simulink model "ReformerSpaceTime"  (R2021a)
settings: Solver=ode23tb  StartTime=0.0  StopTime=10000  RelTol=1e-3
values from neighbouring files (symbols this model uses):
  c0 = zeros(Nx,1)    [init_ReformerSpaceTime.m]
  Nx = 25    [init_ReformerSpaceTime.m]
  p = []    [init_ReformerSpaceTime.m]
settings Model: Creator=djoroya  LastModifiedBy=djoroya
settings DebuggingCC: UnconnectedInputMsg=none  UnconnectedOutputMsg=none  UnconnectedLineMsg=none

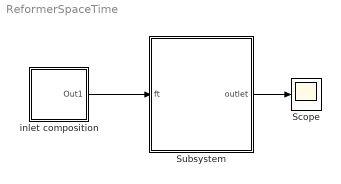
== system ReformerSpaceTime ==
  Scope : Scope
  Subsystem : Subsystem
  inlet composition : Subsystem
  wires:
  inlet composition/1(Out1) -> Subsystem/1(ft)
  Subsystem/1(outlet) -> Scope/1

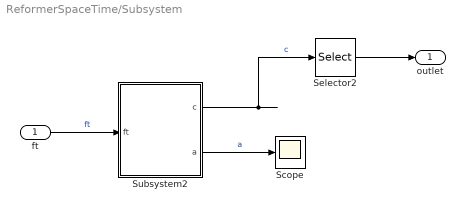
== system ReformerSpaceTime/Subsystem ==
  ft : Inport
  Scope : Scope
  Selector2 : Selector  NumberOfDimensions=2  InputPortWidth=2  IndexOptions=Index vector (dialog),Select all  Indices=Nx,1  OutputSizes=1,1
  Subsystem2 : Subsystem
  outlet : Outport
  wires:
  ft/1 -> Subsystem2/1(ft)  "ft"
  Subsystem2/2(a) -> Scope/1  "a"
  Subsystem2/1(c) -> Selector2/1  "c"
  Selector2/1 -> outlet/1

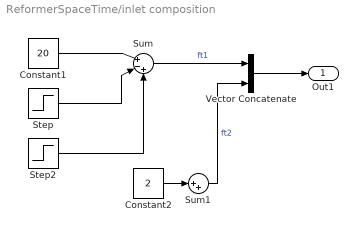
== system ReformerSpaceTime/inlet composition ==
  Constant1 : Constant  Value=20
  Constant2 : Constant  Value=2
  Step : Step  Time=6000  After=20  SampleTime=0
  Step2 : Step  Time=3000  After=10  SampleTime=0
  Sum : Sum  Inputs=|+-+
  Sum1 : Sum  Inputs=|++
  Vector Concatenate : Concatenate  Mode=Multidimensional array  ConcatenateDimension=2
  Out1 : Outport
  wires:
  Constant1/1 -> Sum/1
  Constant2/1 -> Sum1/1
  Sum1/1 -> Vector Concatenate/2  "ft2"
  Sum/1 -> Vector Concatenate/1  "ft1"
  Vector Concatenate/1 -> Out1/1
  Step/1 -> Sum/2
  Step2/1 -> Sum/3

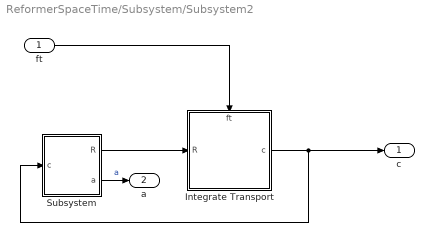
== system ReformerSpaceTime/Subsystem/Subsystem2 ==
  ft : Inport
  Integrate Transport : Subsystem
      settings: PortSchema="{\"entries\":[{\"content\":{\"sides\":[{\"content\":{\"connectorIds\":[\"In1\"]},\"type\":\"ConnectorPlacement.EquallySpacedRectSide\",\"uuid\":\"e3e01424-637b-4a00-a2de-d40794d2ff76\"},{\"content\":{\"connectorIds\":[\"Out1\"],\"side\":\"RIGHT\"},\"type\":\"ConnectorPlacement.EquallySpacedRectSide\",\"uuid\":\"276261e1-850f-4b68-9985-ea5629fd55a5\"},{\"content\":{\"connectorIds\":[\"In2\"],\"side\":\"TOP\"},\"type\":\"ConnectorPlacement.EquallySpacedRectSide\",\"uuid\":\"07b53658-fce3-4297-a7f0-8888709701c4\"}]},\"type\":\"ConnectorPlacement.EquallySpacedConnector\",\"uuid\":\"2f7db6b4-a935-4b8f-9ad3-e9b0cbcdf802\"}],\"packageUris\":[\"http://schema.mathworks.com/mf0/Connector/R2020b\"],\"version\":\"1.0\"}"
  Subsystem : Subsystem
  c : Outport
  a : Outport  Port=2
  wires:
  Subsystem/2(a) -> a/1  "a"
  Subsystem/1(R) -> Integrate Transport/1(R)
  ft/1 -> Integrate Transport/2(ft)
  Integrate Transport/1(c) -> Subsystem/1(c), c/1

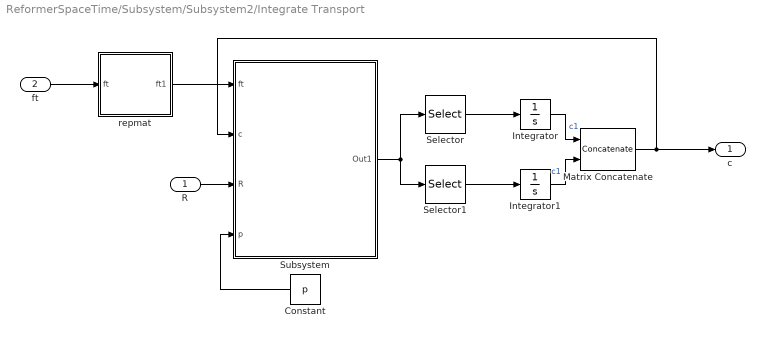
== system ReformerSpaceTime/Subsystem/Subsystem2/Integrate Transport ==
  R : Inport
  ft : Inport  Port=2
  Constant : Constant  Value=p  OutDataTypeStr=Bus: params  LockScale=on
  Integrator : Integrator  InitialCondition=c0
  Integrator1 : Integrator  InitialCondition=c0
  Matrix Concatenate : Concatenate  Mode=Multidimensional array  ConcatenateDimension=2
  Selector : Selector  NumberOfDimensions=2  InputPortWidth=3  IndexOptions=Select all,Index vector (dialog)  Indices=[1 3],1  OutputSizes=1,1
  Selector1 : Selector  NumberOfDimensions=2  InputPortWidth=3  IndexOptions=Select all,Index vector (dialog)  Indices=[1 3],2  OutputSizes=1,1
  Subsystem : Subsystem
  repmat : Subsystem
  c : Outport
  wires:
  ft/1 -> repmat/1(ft)
  repmat/1(ft1) -> Subsystem/1(ft)
  R/1 -> Subsystem/3(R)
  Constant/1 -> Subsystem/4(p)
  Subsystem/1(Out1) -> Selector/1, Selector1/1
  Selector/1 -> Integrator/1
  Selector1/1 -> Integrator1/1
  Integrator/1 -> Matrix Concatenate/1  "c1"
  Integrator1/1 -> Matrix Concatenate/2  "c1"
  Matrix Concatenate/1 -> Subsystem/2(c), c/1

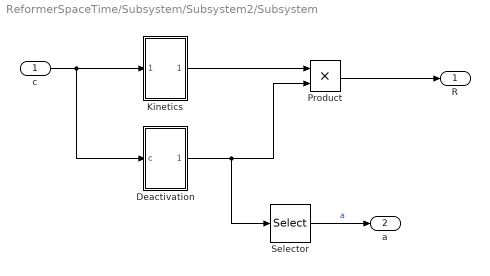
== system ReformerSpaceTime/Subsystem/Subsystem2/Subsystem ==
  c : Inport
  Deactivation : Subsystem
  Kinetics : Subsystem
  Product : Product  OutDataTypeStr=Inherit: Same as first input
  Selector : Selector  NumberOfDimensions=2  InputPortWidth=3  IndexOptions=Select all,Index vector (dialog)  Indices=1,1  OutputSizes=1,1
  R : Outport
  a : Outport  Port=2
  wires:
  c/1 -> Kinetics/1(In1), Deactivation/1(c)
  Kinetics/1(Out1) -> Product/1
  Product/1 -> R/1
  Deactivation/1(Out1) -> Selector/1, Product/2
  Selector/1 -> a/1  "a"

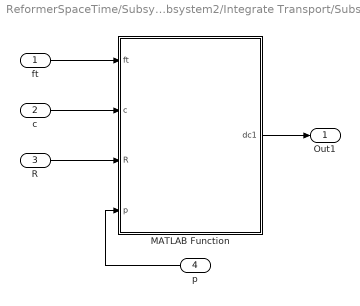
== system ReformerSpaceTime/Subsystem/Subsystem2/Integrate Transport/Subsystem ==
  ft : Inport  PortDimensions=[Nx,2]
  c : Inport  Port=2  PortDimensions=[Nx,2]
  R : Inport  Port=3  PortDimensions=[Nx,2]
  p : Inport  Port=4
  MATLAB Function : MATLAB Function  TreatAsAtomicUnit=on
  Out1 : Outport  PortDimensions=[Nx,2]
  wires:
  MATLAB Function/1(dc1) -> Out1/1
  R/1 -> MATLAB Function/3(R)
  p/1 -> MATLAB Function/4(p)
  c/1 -> MATLAB Function/2(c)
  ft/1 -> MATLAB Function/1(ft)

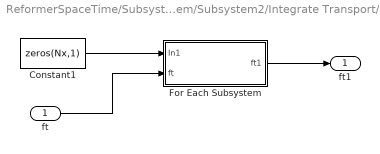
== system ReformerSpaceTime/Subsystem/Subsystem2/Integrate Transport/repmat ==
  ft : Inport
  Constant1 : Constant  Value=zeros(Nx,1)
  For Each Subsystem : Subsystem  TreatAsAtomicUnit=on
  ft1 : Outport
  wires:
  ft/1 -> For Each Subsystem/2(ft)
  For Each Subsystem/1(ft1) -> ft1/1
  Constant1/1 -> For Each Subsystem/1(In1)

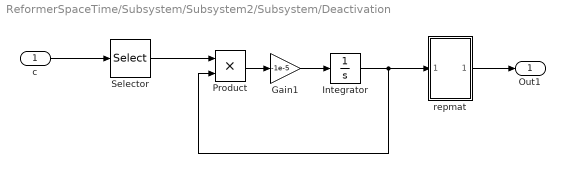
== system ReformerSpaceTime/Subsystem/Subsystem2/Subsystem/Deactivation ==
  c : Inport
  Gain1 : Gain  Gain=-1e-5
  Integrator : Integrator  InitialCondition=ones(Nx,1)
  Product : Product
  Selector : Selector  NumberOfDimensions=2  InputPortWidth=2  IndexOptions=Select all,Index vector (dialog)  Indices=1,1  OutputSizes=1,1
  repmat : Subsystem
  Out1 : Outport
  wires:
  Integrator/1 -> Product/2, repmat/1(In1)
  Product/1 -> Gain1/1
  Gain1/1 -> Integrator/1
  c/1 -> Selector/1
  Selector/1 -> Product/1
  repmat/1(Out1) -> Out1/1

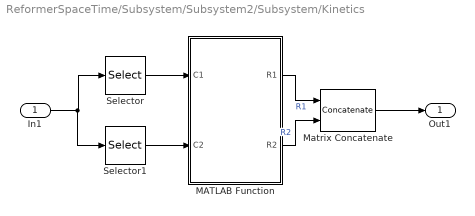
== system ReformerSpaceTime/Subsystem/Subsystem2/Subsystem/Kinetics ==
  In1 : Inport
  MATLAB Function : MATLAB Function  TreatAsAtomicUnit=on
  Matrix Concatenate : Concatenate  Mode=Multidimensional array  ConcatenateDimension=2
  Selector : Selector  NumberOfDimensions=2  InputPortWidth=2  IndexOptions=Select all,Index vector (dialog)  Indices=1,1  OutputSizes=1,1
  Selector1 : Selector  NumberOfDimensions=2  InputPortWidth=2  IndexOptions=Select all,Index vector (dialog)  Indices=2,2  OutputSizes=1,1
  Out1 : Outport
  wires:
  MATLAB Function/2(R2) -> Matrix Concatenate/2  "R2"
  Matrix Concatenate/1 -> Out1/1
  MATLAB Function/1(R1) -> Matrix Concatenate/1  "R1"
  Selector/1 -> MATLAB Function/1(C1)
  Selector1/1 -> MATLAB Function/2(C2)
  In1/1 -> Selector1/1, Selector/1

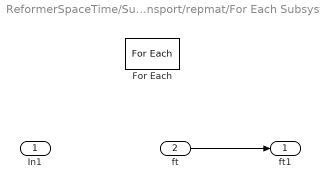
== system ReformerSpaceTime/Subsystem/Subsystem2/Integrate Transport/repmat/For Each Subsystem ==
  In1 : Inport  Partition=on  PartitionDimension=1  PartitionWidth=1  PartitionOffset=0
  ft : Inport  Port=2
  For Each : ForEach  DisableCoverage=on
  ft1 : Outport  ConcatenationDimension=1
  wires:
  ft/1 -> ft1/1

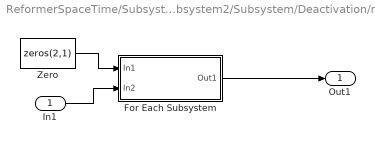
== system ReformerSpaceTime/Subsystem/Subsystem2/Subsystem/Deactivation/repmat ==
  In1 : Inport
  For Each Subsystem : Subsystem  TreatAsAtomicUnit=on
  Zero : Constant  Value=zeros(2,1)  OutDataTypeStr=Inherit: Inherit via back propagation
  Out1 : Outport
  wires:
  For Each Subsystem/1(Out1) -> Out1/1
  In1/1 -> For Each Subsystem/2(In2)
  Zero/1 -> For Each Subsystem/1(In1)

== system ReformerSpaceTime/Subsystem/Subsystem2/Subsystem/Deactivation/repmat/For Each Subsystem ==
  In1 : Inport  Partition=on  PartitionDimension=1  PartitionWidth=1  PartitionOffset=0
  In2 : Inport  Port=2
  For Each : ForEach  DisableCoverage=on
  Out1 : Outport  ConcatenationDimension=2
  wires:
  In2/1 -> Out1/1

== matlab function ReformerSpaceTime/Subsystem/Subsystem2/Subsystem/Kinetics/MATLAB Function ==
  data: C1 input; R1 output; C2 input; R2 output
function [R1,R2] = fcn(C1,C2)
% 
R1 = -C1;
R2 =  C1;
%
% alpha = 1;
% C1_eq = 10;
% C2_eq = 10;
% R1 = alpha*(C1_eq  - C1);
% R2 = alpha*(C2_eq  - C2);

== matlab function ReformerSpaceTime/Subsystem/Subsystem2/Integrate Transport/Subsystem/MATLAB Function ==
  data: ft input; c input; R input; dc1 output; p input
function dc1 = fcn(ft,c,R,p)

dx = p.dx;
Dc = p.Dc;
bc = p.bc;

dc1 = -(1/dx)*(Dc*c + ft.*bc) + R;
